simulink model "Sri_Lanka_S_FINAL_set_points"  (R2024a)
settings: Solver=ode15s  StartTime=0.0  StopTime=600  MaxStep=0.01  RelTol=1e-3
StartFcn:
  | Pref_Set_LAK
  | Pref_set_samanala
  | Pref_Set_UTH
  | Pref_Set_RTB
  | Pref_Set_BWT
  | Pref_Set_UKU
  | Pref_Set_SOBA_GT
  | Pref_Set_SOBA_ST
  | Pref_Set_NLX
  | Pref_Set_YUGA
  | Pref_Set_POL
  | Pref_Set_SOBA_GT
  | Pref_Set_CAN
  | Pref_Set_WIM
  | Pref_Set_BRO
  | Pref_Set_UMA
  | Pref_Set_KUK
  | Pref_Set_VIC
  | Pref_Set_KOT
  | Pref_Set_UKT
  | Pref_Set_BAR
  | Pref_set_KEL_UNIT1
  | Pref_set_KEL_UNIT2
  | Pref_set_KEL_UNIT3
  | Pref_Set_OLX_1
  | Pref_Set_OLX_2
  | Pref_Set_UnitA
  | Pref_Set_UnitB
undefined symbols (not defined in the file): BAR_R, BAR_T_ACT, BAR_Unit_S_nom, BRO_R_P, BRO_R_T, BRO_T_G, BRO_T_R, BRO_T_W, BRO_Unit_S_nom, BWT_R_P, BWT_R_T, BWT_T_R, BWT_T_W, BWT_Unit_S_nom, CAN_R_P, CAN_R_T, CAN_T_G, CAN_T_R, CAN_T_W, CAN_Unit_S_nom, D_T, f_base, H_eq, KEL_CC_F_GT, KEL_CC_F_ST, KEL_CC_T_HRSG, KEL_R, KEL_T_CH, KEL_UNIT1_S_nom, KEL_UNIT2_S_nom, KEL_UNIT3_S_nom, KOT_R_P, KOT_R_T, KOT_T_R, KOT_T_W, KOT_Unit_S_nom, KUK_R_P, KUK_R_T, KUK_T_R, KUK_T_W, KUK_Unit_S_nom, LAK_R, LAK_S_nom, LAU_R, LAU_T_FILT, LAU_T_INV, LAU_Unit_S_nom, MAD_R, MAD_T_FILT, MAD_T_INV, MAD_Unit_S_nom, MAN_K_vir, MAN_T_FILT, MAN_T_INV, MAN_Unit_S_nom, NLX_R_P, NLX_R_T, NLX_T_G, NLX_T_R, NLX_T_W ... (+122)
settings Model: Creator=munas  LastModifiedBy=DIMUTHU

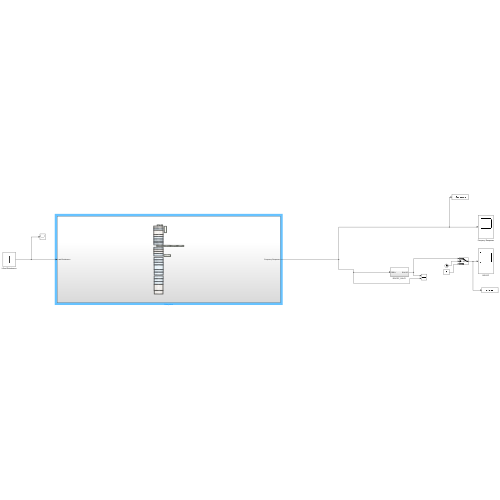
[thumbnail: Simulink's stored preview of the top-level diagram]
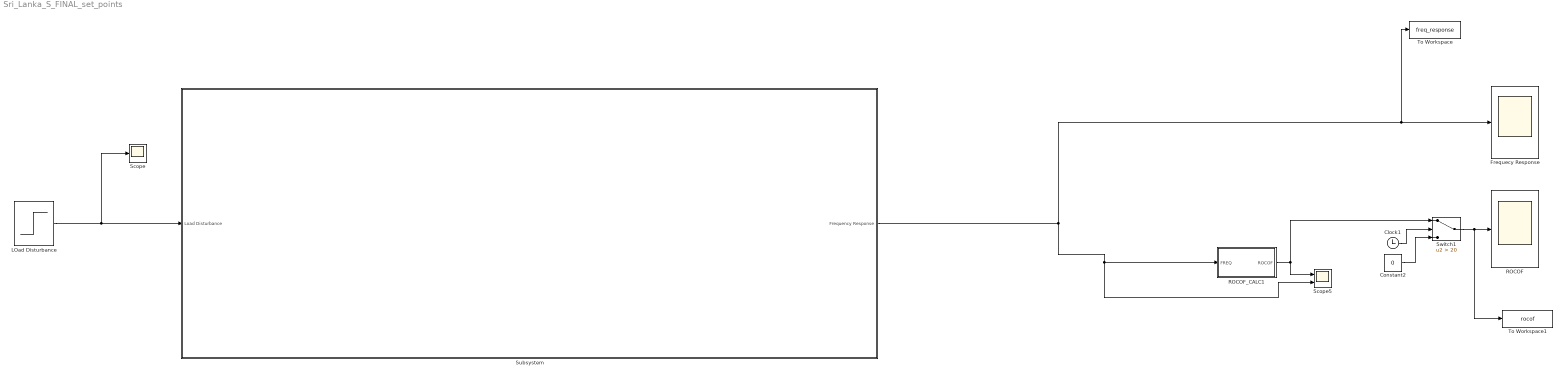
== system Sri_Lanka_S_FINAL_set_points ==
  Clock1 : Clock
  Constant2 : Constant  Value=0
  Frequecy Response : Scope
  LOad Disturbance : Step  Time=t_dist  After=0.05  SampleTime=0
  ROCOF : Scope
  ROCOF_CALC1 : Subsystem
  Scope : Scope
  Scope5 : Scope  NumInputPorts=2
  Subsystem : Subsystem
  Switch1 : Switch  Criteria=u2 > Threshold  Threshold=20  SaturateOnIntegerOverflow=off  InputSameDT=off
  To Workspace : ToWorkspace  VariableName=freq_response  SaveFormat=Timeseries  SampleTime=-1
  To Workspace1 : ToWorkspace  VariableName=rocof  SaveFormat=Timeseries  SampleTime=-1
  wires:
  LOad Disturbance/1 -> Subsystem/1(Load Disturbance), Scope/1
  Subsystem/1(Frequency Response) -> Scope5/2, ROCOF_CALC1/1(FREQ), To Workspace/1, Frequecy Response/1
  Constant2/1 -> Switch1/3
  Switch1/1 -> To Workspace1/1, ROCOF/1
  Clock1/1 -> Switch1/2
  ROCOF_CALC1/1(ROCOF) -> Switch1/1, Scope5/1

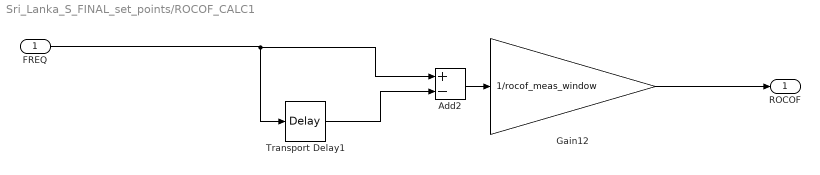
== system Sri_Lanka_S_FINAL_set_points/ROCOF_CALC1 ==
  FREQ : Inport
  Add2 : Sum  Inputs=+-
  Gain12 : Gain  Gain=1/rocof_meas_window
  Transport Delay1 : TransportDelay  DelayTime=rocof_meas_window  InitialOutput=50
  ROCOF : Outport
  wires:
  Transport Delay1/1 -> Add2/2
  Gain12/1 -> ROCOF/1
  Add2/1 -> Gain12/1
  FREQ/1 -> Add2/1, Transport Delay1/1

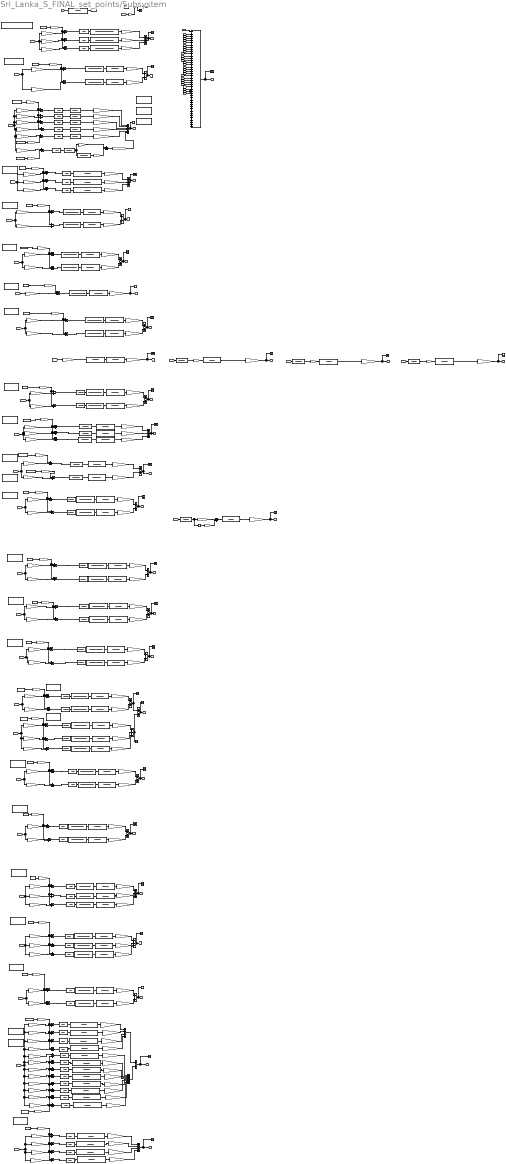
== system Sri_Lanka_S_FINAL_set_points/Subsystem ==
  note: NAYANAJITH
  note: Dinitha
  note: [Steam Turbine Path: 33%]
  note: [Gas Turbine Path: 67%]
  note: SAMANALAWEWA
  note: GRID BLOCK
  note: SUMMING BLOCK
  note: To convert to the frequency
  note: LAKVIJAYA
  note: KELANITISSA
  note: Uthuru Janani plant
  note: RANDENIGALA
  note: RANTAMBE
  note: BOWATENNA
  note: UKUWELA
  note: THAMBAPAVANI WIND FARM: 100 MW
  note: Yugadhanavi GT and ST
  note: New LAXAPANA
  note: Sobadhanavi ST and GT
  note: Polpitiya Plant
  note: Canyon Plant
  note: Wimalasurendra Plant
  note: Kukuleganga Plant
  note: Uma Oya Plant
  note: Old Laxapana Plant
  note: Broadland Plant
  note: Hashan
  note: ANUTHTHARA
  note: Victoria Plant
  note: Upper Kotmale Plant
  note: Kotmale Plant
  note: Colombo Port Barge Plant
  note: Sapugaskanda Plant
  note: Maduru Oya Solar PV subsystem
  note: LAUGFS Hambantota Solar Power Plant
  note: Solar One CeylonSolar Farm
  note: Uppudaluwa Wind Farm
  Load Disturbance : Inport
  " " : TransferFcn  Denominator=[2*H_eq D_T]
  Actuator Delay : TransferFcn  Denominator="[UTH_T_ACT  1]"
  Actuator Delay1 : TransferFcn  Denominator="[UTH_T_ACT  1]"
  Actuator Delay{3..13,15} (12 alike) : TransferFcn  Denominator="[SAP_T_ACT  1]"
  Actuator Delay{14,16..18} (4 alike) : TransferFcn  Denominator="[BAR_T_ACT  1]"
  Actuator Delay2 : TransferFcn  Denominator="[UTH_T_ACT  1]"
  Add{,4,8,13,20..21} (6 alike) : Sum  Inputs=+++
  Add1 : Sum  Inputs=-+++++++++++++++++++++++++++++++++++++++++++
  Add{2,5..7,9..12,14..19,22,25,27..96} (86 alike) : Sum
  Add23 : Sum  Inputs=++++
  Add24 : Sum  Inputs=++++++++
  Add26 : Sum  Inputs=++++
  Add3 : Sum  Inputs=++++++
  Base Scaling Gain : Gain  Gain=SAM_Unit_S_nom / S_base_sys
  Base Scaling Gain GT : Gain  Gain=YUGA_GT_S_nom / S_base_sys
  Base Scaling Gain GT1 : Gain  Gain=YUGA_GT_S_nom / S_base_sys
  Base Scaling Gain GT2 : Gain  Gain=SOBA_GT_S_nom / S_base_sys
  Base Scaling Gain1 : Gain  Gain=SAM_Unit_S_nom / S_base_sys
  Base Scaling Gain10 : Gain  Gain=RTB_Unit_S_nom / S_base_sys
  Base Scaling Gain11 : Gain  Gain=UKU_Unit_S_nom / S_base_sys
  Base Scaling Gain12 : Gain  Gain=BWT_Unit_S_nom / S_base_sys
  Base Scaling Gain13 : Gain  Gain=UKU_Unit_S_nom / S_base_sys
  Base Scaling Gain14 : Gain  Gain=MAN_Unit_S_nom / S_base_sys
  Base Scaling Gain15 : Gain  Gain=SOBA_ST_S_nom/S_base_sys
  Base Scaling Gain16 : Gain  Gain=YUGA_ST_S_nom/S_base_sys
  Base Scaling Gain17 : Gain  Gain=NLX_Unit_S_nom / S_base_sys
  Base Scaling Gain18 : Gain  Gain=NLX_Unit_S_nom / S_base_sys
  Base Scaling Gain19 : Gain  Gain=POL_Unit_S_nom / S_base_sys
  Base Scaling Gain2 : Gain  Gain=RTB_Unit_S_nom / S_base_sys
  Base Scaling Gain20 : Gain  Gain=POL_Unit_S_nom / S_base_sys
  Base Scaling Gain21 : Gain  Gain=WIM_Unit_S_nom / S_base_sys
  Base Scaling Gain22 : Gain  Gain=WIM_Unit_S_nom / S_base_sys
  Base Scaling Gain23 : Gain  Gain=BRO_Unit_S_nom / S_base_sys
  Base Scaling Gain24 : Gain  Gain=BRO_Unit_S_nom / S_base_sys
  Base Scaling Gain25 : Gain  Gain=OLX_Unit_S_nom_1 / S_base_sys
  Base Scaling Gain26 : Gain  Gain=OLX_Unit_S_nom_1 / S_base_sys
  Base Scaling Gain27 : Gain  Gain=OLX_Unit_S_nom_2 / S_base_sys
  Base Scaling Gain28 : Gain  Gain=OLX_Unit_S_nom_2 / S_base_sys
  Base Scaling Gain29 : Gain  Gain=OLX_Unit_S_nom_2 / S_base_sys
  Base Scaling Gain{3..6} (4 alike) : Gain  Gain=KEL_UNIT1_S_nom/ S_base_sys
  Base Scaling Gain30 : Gain  Gain=UMA_Unit_S_nom / S_base_sys
  Base Scaling Gain31 : Gain  Gain=UMA_Unit_S_nom / S_base_sys
  Base Scaling Gain32 : Gain  Gain=KUK_Unit_S_nom / S_base_sys
  Base Scaling Gain33 : Gain  Gain=KUK_Unit_S_nom / S_base_sys
  Base Scaling Gain34 : Gain  Gain=CAN_Unit_S_nom / S_base_sys
  Base Scaling Gain35 : Gain  Gain=CAN_Unit_S_nom / S_base_sys
  Base Scaling Gain36 : Gain  Gain=VIC_Unit_S_nom / S_base_sys
  Base Scaling Gain37 : Gain  Gain=VIC_Unit_S_nom / S_base_sys
  Base Scaling Gain38 : Gain  Gain=VIC_Unit_S_nom / S_base_sys
  Base Scaling Gain39 : Gain  Gain=KOT_Unit_S_nom / S_base_sys
  Base Scaling Gain40 : Gain  Gain=KOT_Unit_S_nom / S_base_sys
  Base Scaling Gain41 : Gain  Gain=UKT_Unit_S_nom / S_base_sys
  Base Scaling Gain42 : Gain  Gain=UKT_Unit_S_nom / S_base_sys
  Base Scaling Gain43 : Gain  Gain=KOT_Unit_S_nom / S_base_sys
  Base Scaling Gain44 : Gain  Gain=MAD_Unit_S_nom / S_base_sys
  Base Scaling Gain45 : Gain  Gain=LAU_Unit_S_nom / S_base_sys
  Base Scaling Gain46 : Gain  Gain=SOC_Unit_S_nom / S_base_sys
  Base Scaling Gain47 : Gain  Gain=UPP_Unit_S_nom / S_base_sys
  Base Scaling Gain7 : Gain  Gain=KEL_UNIT2_S_nom/ S_base_sys
  Base Scaling Gain8 : Gain  Gain=RAN_Unit_S_nom / S_base_sys
  Base Scaling Gain9 : Gain  Gain=RAN_Unit_S_nom / S_base_sys
  Combustr : TransferFcn  Denominator="[KEL_T_CH  1]"
  Constant : Constant  Value=f_base
  Constant1 : Constant  Value=Pref_set_samanala
  Constant10 : Constant  Value=Pref_Set_SOBA_GT
  Constant11 : Constant  Value=Pref_Set_POL
  Constant12 : Constant  Value=Pref_Set_CAN
  Constant13 : Constant  Value=Pref_Set_WIM
  Constant14 : Constant  Value=Pref_Set_BRO
  Constant15 : Constant  Value=Pref_Set_UMA
  Constant16 : Constant  Value=Pref_Set_KUK
  Constant17 : Constant  Value=Pref_Set_VIC
  Constant18 : Constant  Value=Pref_Set_KOT
  Constant19 : Constant  Value=Pref_Set_UKT
  Constant2 : Constant  Value=Pref_Set_LAK
  Constant20 : Constant  Value=Pref_Set_BAR
  Constant21 : Constant  Value=Pref_Set_SOBA_ST
  Constant22 : Constant  Value=Pref_set_KEL_UNIT1
  Constant23 : Constant  Value=Pref_set_KEL_UNIT2
  Constant24 : Constant  Value=Pref_set_KEL_UNIT3
  Constant25 : Constant  Value=Pref_Set_OLX_1
  Constant26 : Constant  Value=Pref_Set_OLX_2
  Constant27 : Constant  Value=Pref_Set_UnitA
  Constant28 : Constant  Value=Pref_Set_UnitB
  Constant3 : Constant  Value=Pref_Set_UTH
  Constant4 : Constant  Value=Pref_Set_RAN
  Constant5 : Constant  Value=Pref_Set_RTB
  Constant6 : Constant  Value=Pref_Set_BWT
  Constant7 : Constant  Value=Pref_Set_UKU
  Constant8 : Constant  Value=Pref_Set_NLX
  Constant9 : Constant  Value=Pref_Set_YUGA
  Derivative : Derivative
  Gain : Gain  Gain=1 / MAD_R
  Gain1 : Gain  Gain=KEL_CC_F_ST
  Gain{8..35} (28 alike) : Gain  Gain=1e6/S_base_sys
  Gain2 : Gain  Gain=KEL_UNIT3_S_nom/ S_base_sys
  Gain3 : Gain  Gain=f_base
  Gain4 : Gain  Gain=1 / LAU_R
  Gain5 : Gain  Gain=1 / SOC_R
  Gain6 : Gain  Gain=1 / UPP_R_P
  Gain7 : Gain  Gain=UPP_K_vir
  Governer{,1..13} (14 alike) : TransferFcn  Denominator=[T_G 1]
  Governer {1..2,7,9,11,13,15,17..19,30..33,35..46} (26 alike) : TransferFcn  Denominator=[T_G 1]
  Governer {8,10,12,14,16} (5 alike) : TransferFcn  Denominator="[KEL_T_CH  1]"
  Governer 20 : TransferFcn  Denominator=[CAN_T_G 1]
  Governer 21 : TransferFcn  Denominator="[WIM_T_G  1]"
  Governer 22 : TransferFcn  Denominator="[WIM_T_G  1]"
  Governer 23 : TransferFcn  Denominator="[BRO_T_G  1]"
  Governer 24 : TransferFcn  Denominator="[BRO_T_G  1]"
  Governer {25..29} (5 alike) : TransferFcn  Denominator="[OLX_T_G  1]"
  Governer 3 : TransferFcn  Denominator=[POL_T_G 1]
  Governer 34 : TransferFcn  Denominator="[CAN_T_G  1]"
  Governer 4 : TransferFcn  Denominator=[POL_T_G 1]
  Governer 5 : TransferFcn  Denominator=[NLX_T_G 1]
  Governer 6 : TransferFcn  Denominator=[NLX_T_G 1]
  Governer GT : TransferFcn  Denominator=[YUGA_GT_T_G 1]
  Governer GT1 : TransferFcn  Denominator=[YUGA_GT_T_G 1]
  Governer GT2 : TransferFcn  Denominator=[SOBA_GT_T_g 1]
  Governer ST : TransferFcn  Denominator=[YUGA_ST_T_ch 1]
  Governer ST1 : TransferFcn  Denominator=[SOBA_ST_T_ch 1]
  HRSG Delay : TransferFcn  Denominator="[KEL_CC_T_HRSG  1]"
  Inverter Delay : TransferFcn  Denominator="[MAN_T_INV  1]"
  Inverter Delay1 : TransferFcn  Denominator=[MAD_T_INV 1]
  Inverter Delay2 : TransferFcn  Denominator=[LAU_T_INV 1]
  Inverter Delay3 : TransferFcn  Denominator=[SOC_T_INV 1]
  Inverter Delay4 : TransferFcn  Denominator=[UPP_T_INV 1]
  PLL Filter : TransferFcn  Denominator=[LAU_T_FILT 1]
  PLL Filter1 : TransferFcn  Denominator=[SOC_T_FILT 1]
  PURE DROOP : Gain  Gain=-1/LAK_R
  PURE DROOP GT : Gain  Gain=-1/YUGA_GT_R
  PURE DROOP GT1 : Gain  Gain=-1/YUGA_GT_R
  PURE DROOP GT2 : Gain  Gain=-1/SOBA_GT_R
  PURE DROOP ST : Gain  Gain=-1/YUGA_ST_R
  PURE DROOP ST1 : Gain  Gain=-1/SOBA_ST_R
  PURE DROOP1 : Gain  Gain=-1/LAK_R
  PURE DROOP{6..11} (6 alike) : Gain  Gain=-1/KEL_R
  PURE DROOP12 : Gain  Gain=-1/UTH_R
  PURE DROOP13 : Gain  Gain=-1/UTH_R
  PURE DROOP14 : Gain  Gain=-1/UTH_R
  PURE DROOP15 : Gain  Gain=-1/RAN_R_P
  PURE DROOP16 : Gain  Gain=-1/RAN_R_P
  PURE DROOP17 : Gain  Gain=-1/RTB_R_P
  PURE DROOP18 : Gain  Gain=-1/UKU_R_P
  PURE DROOP19 : Gain  Gain=-1/BWT_R_P
  PURE DROOP2 : Gain  Gain=-1/LAK_R
  PURE DROOP20 : Gain  Gain=-1/UKU_R_P
  PURE DROOP21 : Gain  Gain=-1/BWT_R_P
  PURE DROOP22 : Gain  Gain=-1/NLX_R_P
  PURE DROOP23 : Gain  Gain=-1/NLX_R_P
  PURE DROOP24 : Gain  Gain=-1/POL_R_P
  PURE DROOP25 : Gain  Gain=-1/POL_R_P
  PURE DROOP26 : Gain  Gain=-1/CAN_R_P
  PURE DROOP27 : Gain  Gain=-1/WIM_R_P
  PURE DROOP28 : Gain  Gain=-1/WIM_R_P
  PURE DROOP29 : Gain  Gain=-1/BRO_R_P
  PURE DROOP3 : Gain  Gain=-1/SAM_R_P
  PURE DROOP30 : Gain  Gain=-1/BRO_R_P
  PURE DROOP{31..35} (5 alike) : Gain  Gain=-1/OLX_R_P
  PURE DROOP36 : Gain  Gain=-1/UMA_R_P
  PURE DROOP37 : Gain  Gain=-1/UMA_R_P
  PURE DROOP38 : Gain  Gain=-1/KUK_R_P
  PURE DROOP39 : Gain  Gain=-1/KUK_R_P
  PURE DROOP4 : Gain  Gain=-1/SAM_R_P
  PURE DROOP40 : Gain  Gain=-1/CAN_R_P
  PURE DROOP41 : Gain  Gain=-1/VIC_R_P
  PURE DROOP42 : Gain  Gain=-1/VIC_R_P
  PURE DROOP43 : Gain  Gain=-1/VIC_R_P
  PURE DROOP44 : Gain  Gain=-1/KOT_R_P
  PURE DROOP45 : Gain  Gain=-1/KOT_R_P
  PURE DROOP46 : Gain  Gain=-1/UKT_R_P
  PURE DROOP47 : Gain  Gain=-1/UKT_R_P
  PURE DROOP48 : Gain  Gain=-1/KOT_R_P
  PURE DROOP{49..60} (12 alike) : Gain  Gain=-1/SAP_R
  PURE DROOP5 : Gain  Gain=-1/RTB_R_P
  PURE DROOP{61..64} (4 alike) : Gain  Gain=-1/BAR_R
  Scaling : Sum
  Scaling 1 : Gain  Gain=LAK_S_nom / S_base_sys
  Scaling {7..10} (4 alike) : Gain  Gain=SAP_A_Unit_S_nom / S_base_sys
  Scaling {11..18} (8 alike) : Gain  Gain=SAP_B_Unit_S_nom / S_base_sys
  Scaling {19..22} (4 alike) : Gain  Gain=BAR_Unit_S_nom / S_base_sys
  Scaling 2 : Gain  Gain=LAK_S_nom / S_base_sys
  Scaling 3 : Gain  Gain=LAK_S_nom / S_base_sys
  Scaling 4 : Gain  Gain=UTH_Unit_S_nom / S_base_sys
  Scaling 5 : Gain  Gain=UTH_Unit_S_nom / S_base_sys
  Scaling 6 : Gain  Gain=UTH_Unit_S_nom / S_base_sys
  Scope{,1..31} (32 alike) : Scope
  Slider : SliderBlock  ScaleMax=300
  Slider1 : SliderBlock  ScaleMax=60
  Slider10 : SliderBlock  ScaleMax=130
  Slider11 : SliderBlock  ScaleMax=45
  Slider12 : SliderBlock  ScaleMax=30
  Slider13 : SliderBlock  ScaleMax=25
  Slider14 : SliderBlock  ScaleMax=17.5
  Slider15 : SliderBlock  ScaleMax=60
  Slider16 : SliderBlock  ScaleMax=40
  Slider17 : SliderBlock  ScaleMax=70
  Slider18 : SliderBlock  ScaleMax=67
  Slider19 : SliderBlock  ScaleMax=83
  Slider2 : SliderBlock  ScaleMax=8
  Slider20 : SliderBlock  ScaleMax=15
  Slider21 : SliderBlock  ScaleMax=20
  Slider22 : SliderBlock  ScaleMax=115
  Slider23 : SliderBlock  ScaleMax=165
  Slider24 : SliderBlock  ScaleMax=12.5
  Slider25 : SliderBlock  ScaleMax=8.33
  Slider26 : SliderBlock  ScaleMax=20
  Slider27 : SliderBlock  ScaleMax=10
  Slider3 : SliderBlock  ScaleMax=63
  Slider4 : SliderBlock  ScaleMax=26
  Slider5 : SliderBlock  ScaleMax=40
  Slider6 : SliderBlock  ScaleMax=20
  Slider7 : SliderBlock  ScaleMax=50
  Slider8 : SliderBlock
  Slider9 : SliderBlock  ScaleMax=220
  Sum : Sum  Inputs=|++
  Synthetic Inertia : TransferFcn  Numerator="[MAN_K_vir  0]"  Denominator="[MAN_T_FILT  1]"
  Transfer Fcn : TransferFcn  Denominator=[MAD_T_FILT 1]
  Transfer Fcn1 : TransferFcn  Denominator=[UPP_T_FILT 1]
  Transient Droop : TransferFcn  Numerator="[SAM_T_R  1]"  Denominator="[SAM_T_R*(SAM_R_T/SAM_R_P)  1]"
  Transient Droop GT : TransferFcn  Denominator="[YUGA_GT_T_t  1]"
  Transient Droop GT1 : TransferFcn  Denominator="[YUGA_GT_T_t  1]"
  Transient Droop GT2 : TransferFcn  Denominator="[SOBA_GT_T_t  1]"
  Transient Droop ST : TransferFcn  Denominator="[YUGA_ST_T_hrsga  1]"
  Transient Droop ST1 : TransferFcn  Denominator="[SOBA_ST_T_hrsga  1]"
  Transient Droop1 : TransferFcn  Numerator="[SAM_T_R  1]"  Denominator="[SAM_T_R*(SAM_R_T/SAM_R_P)  1]"
  Transient Droop10 : TransferFcn  Numerator="[NLX_T_R  1]"  Denominator="[NLX_T_R*(NLX_R_T/NLX_R_P)  1]"
  Transient Droop11 : TransferFcn  Numerator=[POL_T_R 1]  Denominator="[POL_T_R*(POL_R_T/POL_R_P)  1]"
  Transient Droop12 : TransferFcn  Numerator="[POL_T_R  1]"  Denominator="[POL_T_R*(POL_R_T/POL_R_P)  1]"
  Transient Droop13 : TransferFcn  Numerator=[BRO_T_R 1]  Denominator="[BRO_T_R*(BRO_R_T/BRO_R_P)  1]"
  Transient Droop14 : TransferFcn  Numerator=[BRO_T_R 1]  Denominator="[BRO_T_R*(BRO_R_T/BRO_R_P)  1]"
  Transient Droop{15..19} (5 alike) : TransferFcn  Numerator=[OLX_T_R 1]  Denominator="[OLX_T_R*(OLX_R_T/OLX_R_P)  1]"
  Transient Droop2 : TransferFcn  Numerator="[RAN_T_R  1]"  Denominator="[(RAN_R_T / RAN_R_P) * RAN_T_R   1]"
  Transient Droop20 : TransferFcn  Numerator="[UMA_T_R  1]"  Denominator="[UMA_T_R*(UMA_R_T/UMA_R_P)  1]"
  Transient Droop21 : TransferFcn  Numerator="[UMA_T_R  1]"  Denominator="[UMA_T_R*(UMA_R_T/UMA_R_P)  1]"
  Transient Droop22 : TransferFcn  Numerator="[KUK_T_R  1]"  Denominator="[KUK_T_R*(KUK_R_T/KUK_R_P)  1]"
  Transient Droop23 : TransferFcn  Numerator="[KUK_T_R  1]"  Denominator="[KUK_T_R*(KUK_R_T/KUK_R_P)  1]"
  Transient Droop24 : TransferFcn  Numerator=[CAN_T_R 1]  Denominator="[CAN_T_R*(CAN_R_T/CAN_R_P)  1]"
  Transient Droop25 : TransferFcn  Numerator=[CAN_T_R 1]  Denominator="[CAN_T_R*(CAN_R_T/CAN_R_P)  1]"
  Transient Droop26 : TransferFcn  Numerator=[WIM_T_R 1]  Denominator="[WIM_T_R*(WIM_R_T/WIM_R_P)  1]"
  Transient Droop27 : TransferFcn  Numerator=[WIM_T_R 1]  Denominator="[WIM_T_R*(WIM_R_T/WIM_R_P)  1]"
  Transient Droop28 : TransferFcn  Numerator="[VIC_T_R  1]"  Denominator="[VIC_T_R*(VIC_R_T/VIC_R_P)  1]"
  Transient Droop29 : TransferFcn  Numerator="[VIC_T_R  1]"  Denominator="[VIC_T_R*(VIC_R_T/VIC_R_P)  1]"
  Transient Droop3 : TransferFcn  Numerator="[RAN_T_R  1]"  Denominator="[(RAN_R_T / RAN_R_P) * RAN_T_R   1]"
  Transient Droop30 : TransferFcn  Numerator="[VIC_T_R  1]"  Denominator="[VIC_T_R*(VIC_R_T/VIC_R_P)  1]"
  Transient Droop31 : TransferFcn  Numerator="[KOT_T_R  1]"  Denominator="[KOT_T_R*(KOT_R_T/KOT_R_P)  1]"
  Transient Droop32 : TransferFcn  Numerator="[KOT_T_R  1]"  Denominator="[KOT_T_R*(KOT_R_T/KOT_R_P)  1]"
  Transient Droop33 : TransferFcn  Numerator="[UKT_T_R  1]"  Denominator="[UKT_T_R*(UKT_R_T/UKT_R_P)  1]"
  Transient Droop34 : TransferFcn  Numerator="[UKT_T_R  1]"  Denominator="[UKT_T_R*(UKT_R_T/UKT_R_P)  1]"
  Transient Droop35 : TransferFcn  Numerator="[KOT_T_R  1]"  Denominator="[KOT_T_R*(KOT_R_T/KOT_R_P)  1]"
  Transient Droop4 : TransferFcn  Numerator="[RTB_T_R  1]"  Denominator="[(RTB_R_T / RTB_R_P) * RTB_T_R   1]"
  Transient Droop5 : TransferFcn  Numerator="[RTB_T_R  1]"  Denominator="[(RTB_R_T / RTB_R_P) * RTB_T_R   1]"
  Transient Droop6 : TransferFcn  Numerator="[BWT_T_R  1]"  Denominator="[(BWT_R_T / BWT_R_P) * BWT_T_R   1]"
  Transient Droop7 : TransferFcn  Numerator="[UKU_T_R  1]"  Denominator="[(UKU_R_T / UKU_R_P) * UKU_T_R   1]"
  Transient Droop8 : TransferFcn  Numerator="[UKU_T_R  1]"  Denominator="[(UKU_R_T / UKU_R_P) * UKU_T_R   1]"
  Transient Droop9 : TransferFcn  Numerator=[NLX_T_R 1]  Denominator="[NLX_T_R*(NLX_R_T/NLX_R_P)  1]"
  Turbine Dynamics (Reheat) : TransferFcn  Numerator="[RHT_F_HP*RHT_T_RH  1]"  Denominator="[RHT_T_CH*RHT_T_RH  (RHT_T_CH+RHT_T_RH)  1]"
  Turbine Dynamics (Reheat)1 : TransferFcn  Numerator="[RHT_F_HP*RHT_T_RH  1]"  Denominator="[RHT_T_CH*RHT_T_RH  (RHT_T_CH+RHT_T_RH)  1]"
  Turbine Dynamics (Reheat)2 : TransferFcn  Numerator="[RHT_F_HP*RHT_T_RH  1]"  Denominator="[RHT_T_CH*RHT_T_RH  (RHT_T_CH+RHT_T_RH)  1]"
  Water Column : TransferFcn  Numerator="[-SAM_T_W  1]"  Denominator="[0.5*SAM_T_W  1]"
  Water Column1 : TransferFcn  Numerator="[-SAM_T_W  1]"  Denominator="[0.5*SAM_T_W  1]"
  Water Column10 : TransferFcn  Numerator="[-NLX_T_W  1]"  Denominator="[0.5*NLX_T_W  1]"
  Water Column11 : TransferFcn  Numerator="[-POL_T_W  1]"  Denominator="[0.5*POL_T_W  1]"
  Water Column12 : TransferFcn  Numerator="[-POL_T_W  1]"  Denominator="[0.5*POL_T_W  1]"
  Water Column13 : TransferFcn  Numerator="[-BRO_T_W  1]"  Denominator="[0.5*BRO_T_W  1]"
  Water Column14 : TransferFcn  Numerator="[-BRO_T_W  1]"  Denominator="[0.5*BRO_T_W  1]"
  Water Column{15..19} (5 alike) : TransferFcn  Numerator="[-OLX_T_W  1]"  Denominator="[0.5*OLX_T_W  1]"
  Water Column2 : TransferFcn  Numerator="[-RAN_T_W  1]"  Denominator="[0.5 * RAN_T_W   1]"
  Water Column20 : TransferFcn  Numerator="[-UMA_T_W  1]"  Denominator="[0.5*UMA_T_W  1]"
  Water Column21 : TransferFcn  Numerator="[-UMA_T_W  1]"  Denominator="[0.5*UMA_T_W  1]"
  Water Column22 : TransferFcn  Numerator="[-KUK_T_W  1]"  Denominator="[0.5*KUK_T_W  1]"
  Water Column23 : TransferFcn  Numerator="[-KUK_T_W  1]"  Denominator="[0.5*KUK_T_W  1]"
  Water Column24 : TransferFcn  Numerator="[-CAN_T_W  1]"  Denominator="[0.5*CAN_T_W  1]"
  Water Column25 : TransferFcn  Numerator="[-CAN_T_W  1]"  Denominator="[0.5*CAN_T_W  1]"
  Water Column26 : TransferFcn  Numerator="[-WIM_T_W  1]"  Denominator="[0.5*WIM_T_W  1]"
  Water Column27 : TransferFcn  Numerator="[-WIM_T_W  1]"  Denominator="[0.5*WIM_T_W  1]"
  Water Column28 : TransferFcn  Numerator="[-VIC_T_W  1]"  Denominator="[0.5*VIC_T_W  1]"
  Water Column29 : TransferFcn  Numerator="[-VIC_T_W  1]"  Denominator="[0.5*VIC_T_W  1]"
  Water Column3 : TransferFcn  Numerator="[-RAN_T_W  1]"  Denominator="[0.5 * RAN_T_W   1]"
  Water Column30 : TransferFcn  Numerator="[-VIC_T_W  1]"  Denominator="[0.5*VIC_T_W  1]"
  Water Column31 : TransferFcn  Numerator="[-KOT_T_W  1]"  Denominator="[0.5*KOT_T_W  1]"
  Water Column32 : TransferFcn  Numerator="[-KOT_T_W  1]"  Denominator="[0.5*KOT_T_W  1]"
  Water Column33 : TransferFcn  Numerator="[-UKT_T_W  1]"  Denominator="[0.5*UKT_T_W  1]"
  Water Column34 : TransferFcn  Numerator="[-UKT_T_W  1]"  Denominator="[0.5*UKT_T_W  1]"
  Water Column35 : TransferFcn  Numerator="[-KOT_T_W  1]"  Denominator="[0.5*KOT_T_W  1]"
  Water Column4 : TransferFcn  Numerator="[-RTB_T_W  1]"  Denominator="[0.5 * RTB_T_W   1]"
  Water Column5 : TransferFcn  Numerator="[-RTB_T_W  1]"  Denominator="[0.5 * RTB_T_W   1]"
  Water Column6 : TransferFcn  Numerator="[-BWT_T_W  1]"  Denominator="[0.5 * BWT_T_W   1]"
  Water Column7 : TransferFcn  Numerator="[-UKU_T_W  1]"  Denominator="[0.5 * UKU_T_W   1]"
  Water Column8 : TransferFcn  Numerator="[-UKU_T_W  1]"  Denominator="[0.5 * UKU_T_W   1]"
  Water Column9 : TransferFcn  Numerator="[-NLX_T_W  1]"  Denominator="[0.5*NLX_T_W  1]"
  | Gain: F_GT : Gain  Gain=KEL_CC_F_GT
  Frequency Response : Outport
  wires:
  Governer 1/1 -> Turbine Dynamics (Reheat)/1
  Turbine Dynamics (Reheat)/1 -> Scaling 1/1
  Sum/1 -> Scope2/1, Frequency Response/1
  Constant/1 -> Sum/1
  Scaling 1/1 -> Add/1
  Governer 2/1 -> Turbine Dynamics (Reheat)1/1
  Turbine Dynamics (Reheat)1/1 -> Scaling 2/1
  Scaling 2/1 -> Add/2
  Governer/1 -> Turbine Dynamics (Reheat)2/1
  Turbine Dynamics (Reheat)2/1 -> Scaling 3/1
  Scaling 3/1 -> Add/3
  Add/1 -> Scope3/1, [LAK]
  [P_acc] -> " "/1
  " "/1 -> [Rotor_Dev]
  [Rotor_Dev] -> PURE DROOP2/1, PURE DROOP/1, PURE DROOP1/1
  [Rotor_Dev] -> Gain3/1
  [LAK] -> Add1/2
  Add1/1 -> Scope/1, [P_acc]
  Load Disturbance/1 -> Add1/1
  [Rotor_Dev] -> PURE DROOP3/1, PURE DROOP4/1
  Base Scaling Gain/1 -> Add2/1
  Add2/1 -> Scope1/1, [SAM]
  Transient Droop/1 -> Water Column/1
  Water Column/1 -> Base Scaling Gain/1
  Water Column1/1 -> Base Scaling Gain1/1
  Transient Droop1/1 -> Water Column1/1
  Base Scaling Gain1/1 -> Add2/2
  [SAM] -> Add1/3
  Gain3/1 -> Sum/2
  [Rotor_Dev] -> PURE DROOP8/1, PURE DROOP7/1, PURE DROOP6/1, PURE DROOP11/1, PURE DROOP10/1, PURE DROOP9/1
  Governer 7/1 -> Governer 8/1
  Governer 8/1 -> Base Scaling Gain3/1
  Governer 9/1 -> Governer 10/1
  Governer 10/1 -> Base Scaling Gain4/1
  Governer 11/1 -> Governer 12/1
  Governer 12/1 -> Base Scaling Gain5/1
  Governer 13/1 -> Governer 14/1
  Governer 14/1 -> Base Scaling Gain6/1
  Governer 15/1 -> Governer 16/1
  Governer 16/1 -> Base Scaling Gain7/1
  Governer 17/1 -> Combustr/1
  HRSG Delay/1 -> Gain1/1
  Combustr/1 -> HRSG Delay/1, | Gain: F_GT/1
  | Gain: F_GT/1 -> Scaling/1
  Gain1/1 -> Scaling/2
  Scaling/1 -> Gain2/1
  Base Scaling Gain3/1 -> Add3/1
  Base Scaling Gain4/1 -> Add3/2
  Base Scaling Gain5/1 -> Add3/3
  Base Scaling Gain6/1 -> Add3/4
  Base Scaling Gain7/1 -> Add3/5
  Gain2/1 -> Add3/6
  Add3/1 -> Scope9/1, [KEL]
  [KEL] -> Add1/4
  Actuator Delay2/1 -> Scaling 6/1
  Add4/1 -> Scope4/1, [UTH]
  Scaling 6/1 -> Add4/3
  Governer 19/1 -> Actuator Delay1/1
  Governer1/1 -> Actuator Delay2/1
  Scaling 4/1 -> Add4/1
  [Rotor_Dev] -> PURE DROOP14/1, PURE DROOP13/1, PURE DROOP12/1
  Actuator Delay1/1 -> Scaling 5/1
  Governer 18/1 -> Actuator Delay/1
  Scaling 5/1 -> Add4/2
  Actuator Delay/1 -> Scaling 4/1
  [UTH] -> Add1/5
  [Rotor_Dev] -> PURE DROOP16/1, PURE DROOP15/1
  Transient Droop2/1 -> Water Column2/1
  Base Scaling Gain8/1 -> Add5/1
  Water Column2/1 -> Base Scaling Gain8/1
  Add5/1 -> Scope5/1, [RAN]
  Transient Droop3/1 -> Water Column3/1
  Water Column3/1 -> Base Scaling Gain9/1
  Base Scaling Gain9/1 -> Add5/2
  [RAN] -> Add1/6
  Add6/1 -> Scope6/1, [RTB]
  [Rotor_Dev] -> PURE DROOP17/1, PURE DROOP5/1
  Water Column4/1 -> Base Scaling Gain2/1
  Base Scaling Gain2/1 -> Add6/1
  Base Scaling Gain10/1 -> Add6/2
  Transient Droop4/1 -> Water Column4/1
  [RTB] -> Add1/7
  Transient Droop5/1 -> Water Column5/1
  Water Column5/1 -> Base Scaling Gain10/1
  Transient Droop6/1 -> Water Column6/1
  [Rotor_Dev] -> PURE DROOP19/1
  Water Column6/1 -> Base Scaling Gain12/1
  Base Scaling Gain12/1 -> Scope7/1, [BWT]
  [BWT] -> Add1/8
  Transient Droop7/1 -> Water Column7/1
  Base Scaling Gain13/1 -> Add7/1
  [Rotor_Dev] -> PURE DROOP18/1, PURE DROOP20/1
  Water Column7/1 -> Base Scaling Gain13/1
  Add7/1 -> Scope8/1, [UKU]
  Base Scaling Gain11/1 -> Add7/2
  Water Column8/1 -> Base Scaling Gain11/1
  Transient Droop8/1 -> Water Column8/1
  [UKU] -> Add1/9
  Base Scaling Gain14/1 -> Scope10/1, [MAN]
  Inverter Delay/1 -> Base Scaling Gain14/1
  [Rotor_Dev] -> PURE DROOP21/1
  PURE DROOP21/1 -> Synthetic Inertia/1
  Synthetic Inertia/1 -> Inverter Delay/1
  [MAN] -> Add1/10
  Water Column10/1 -> Base Scaling Gain18/1
  Water Column11/1 -> Base Scaling Gain19/1
  Governer 6/1 -> Transient Droop10/1
  Base Scaling Gain GT2/1 -> Add9/1
  Base Scaling Gain17/1 -> Add10/1
  Transient Droop10/1 -> Water Column10/1
  Governer GT2/1 -> Transient Droop GT2/1
  Add9/1 -> Scope12/1, [SOBA]
  Transient Droop9/1 -> Water Column9/1
  Base Scaling Gain GT/1 -> Add8/1
  Base Scaling Gain15/1 -> Add9/2
  Governer ST/1 -> Transient Droop ST/1
  Transient Droop GT/1 -> Base Scaling Gain GT/1
  [Rotor_Dev] -> PURE DROOP ST/1, PURE DROOP GT1/1, PURE DROOP GT/1
  Base Scaling Gain GT1/1 -> Add8/2
  Transient Droop GT1/1 -> Base Scaling Gain GT1/1
  Governer 3/1 -> Transient Droop11/1
  [Rotor_Dev] -> PURE DROOP25/1, PURE DROOP24/1
  Governer 5/1 -> Transient Droop9/1
  Base Scaling Gain19/1 -> Add11/1
  Base Scaling Gain18/1 -> Add10/2
  Transient Droop GT2/1 -> Base Scaling Gain GT2/1
  Governer GT/1 -> Transient Droop GT/1
  Add8/1 -> Scope11/1, [YUGA]
  Transient Droop ST/1 -> Base Scaling Gain16/1
  Governer 4/1 -> Transient Droop12/1
  [Rotor_Dev] -> PURE DROOP23/1, PURE DROOP22/1
  [Rotor_Dev] -> PURE DROOP ST1/1, PURE DROOP GT2/1
  Add11/1 -> Scope14/1, [POL]
  Base Scaling Gain20/1 -> Add11/2
  Transient Droop ST1/1 -> Base Scaling Gain15/1
  Transient Droop11/1 -> Water Column11/1
  Governer GT1/1 -> Transient Droop GT1/1
  Base Scaling Gain16/1 -> Add8/3
  Add10/1 -> Scope13/1, [NLX]
  Water Column9/1 -> Base Scaling Gain17/1
  Water Column12/1 -> Base Scaling Gain20/1
  Governer ST1/1 -> Transient Droop ST1/1
  Transient Droop12/1 -> Water Column12/1
  [NLX] -> Add1/13
  [YUGA] -> Add1/12
  [SOBA] -> Add1/11
  [POL] -> Add1/14
  Base Scaling Gain33/1 -> Add16/2
  Transient Droop21/1 -> Water Column21/1
  Add14/1 -> Scope18/1, [OLX]
  Governer 29/1 -> Transient Droop19/1
  [Rotor_Dev] -> PURE DROOP39/1, PURE DROOP38/1
  Base Scaling Gain21/1 -> Add18/1
  Governer 27/1 -> Transient Droop18/1
  Base Scaling Gain24/1 -> Add19/2
  Governer 33/1 -> Transient Droop23/1
  Base Scaling Gain32/1 -> Add16/1
  Transient Droop20/1 -> Water Column20/1
  Water Column15/1 -> Base Scaling Gain25/1
  Water Column23/1 -> Base Scaling Gain33/1
  Base Scaling Gain31/1 -> Add15/2
  Governer 26/1 -> Transient Droop15/1
  Base Scaling Gain30/1 -> Add15/1
  Water Column21/1 -> Base Scaling Gain31/1
  Base Scaling Gain28/1 -> Add13/2
  Add15/1 -> Scope19/1, [UMA]
  Governer 30/1 -> Transient Droop20/1
  [Rotor_Dev] -> PURE DROOP31/1, PURE DROOP32/1
  Water Column13/1 -> Base Scaling Gain23/1
  Governer 28/1 -> Transient Droop17/1
  [Rotor_Dev] -> PURE DROOP26/1, PURE DROOP40/1
  [Rotor_Dev] -> PURE DROOP29/1, PURE DROOP30/1
  Transient Droop19/1 -> Water Column19/1
  Add18/1 -> Scope22/1, [WIM]
  Water Column18/1 -> Base Scaling Gain28/1
  Add13/1 -> Add14/2, Scope17/1
  Water Column22/1 -> Base Scaling Gain32/1
  Transient Droop14/1 -> Water Column14/1
  Governer 24/1 -> Transient Droop13/1
  Transient Droop15/1 -> Water Column15/1
  Base Scaling Gain27/1 -> Add13/1
  [Rotor_Dev] -> PURE DROOP35/1, PURE DROOP33/1, PURE DROOP34/1
  Water Column24/1 -> Base Scaling Gain34/1
  Transient Droop22/1 -> Water Column22/1
  Water Column16/1 -> Base Scaling Gain26/1
  Transient Droop18/1 -> Water Column18/1
  Governer 25/1 -> Transient Droop16/1
  Transient Droop17/1 -> Water Column17/1
  Water Column14/1 -> Base Scaling Gain24/1
  Base Scaling Gain22/1 -> Add18/2
  [Rotor_Dev] -> PURE DROOP27/1, PURE DROOP28/1
  Governer 21/1 -> Transient Droop27/1
  Transient Droop16/1 -> Water Column16/1
  Base Scaling Gain29/1 -> Add13/3
  Transient Droop26/1 -> Water Column26/1
  Governer 23/1 -> Transient Droop14/1
  Transient Droop27/1 -> Water Column27/1
  [Rotor_Dev] -> PURE DROOP37/1, PURE DROOP36/1
  Base Scaling Gain23/1 -> Add19/1
  Transient Droop13/1 -> Water Column13/1
  Water Column25/1 -> Base Scaling Gain35/1
  Governer 20/1 -> Transient Droop25/1
  Add19/1 -> Scope15/1, [BRO]
  Transient Droop25/1 -> Water Column25/1
  Water Column17/1 -> Base Scaling Gain27/1
  Base Scaling Gain34/1 -> Add17/1
  Governer 34/1 -> Transient Droop24/1
  Transient Droop24/1 -> Water Column24/1
  Governer 22/1 -> Transient Droop26/1
  Base Scaling Gain26/1 -> Add12/2
  Add16/1 -> Scope20/1, [KUK]
  Base Scaling Gain35/1 -> Add17/2
  Water Column26/1 -> Base Scaling Gain21/1
  Add17/1 -> Scope21/1, [CAN]
  Add12/1 -> Add14/1, Scope16/1
  Governer 32/1 -> Transient Droop22/1
  Governer 31/1 -> Transient Droop21/1
  Water Column27/1 -> Base Scaling Gain22/1
  Water Column20/1 -> Base Scaling Gain30/1
  Transient Droop23/1 -> Water Column23/1
  Water Column19/1 -> Base Scaling Gain29/1
  Base Scaling Gain25/1 -> Add12/1
  [BRO] -> Add1/17
  [WIM] -> Add1/16
  [UMA] -> Add1/19
  [CAN] -> Add1/15
  [KUK] -> Add1/20
  [OLX] -> Add1/18
  Scaling 22/1 -> Add26/4
  Governer13/1 -> Actuator Delay17/1
  Base Scaling Gain37/1 -> Add20/2
  Actuator Delay5/1 -> Scaling 15/1
  Actuator Delay15/1 -> Scaling 16/1
  Actuator Delay14/1 -> Scaling 19/1
  [Rotor_Dev] -> PURE DROOP43/1, PURE DROOP41/1, PURE DROOP42/1
  Governer 35/1 -> Transient Droop28/1
  Scaling 20/1 -> Add26/1
  Scaling 14/1 -> Add24/3
  Water Column33/1 -> Base Scaling Gain41/1
  Water Column32/1 -> Base Scaling Gain40/1
  Scaling 18/1 -> Add24/6
  Scaling 11/1 -> Add24/1
  Water Column30/1 -> Base Scaling Gain38/1
  Actuator Delay10/1 -> Scaling 17/1
  Actuator Delay7/1 -> Scaling 12/1
  Actuator Delay8/1 -> Scaling 13/1
  Scaling 7/1 -> Add23/1
  Scaling 19/1 -> Add26/2
  Actuator Delay4/1 -> Scaling 11/1
  Add22/1 -> Scope25/1, [UKT]
  Scaling 9/1 -> Add23/3
  [Rotor_Dev] -> PURE DROOP48/1, PURE DROOP45/1, PURE DROOP44/1
  Actuator Delay11/1 -> Scaling 9/1
  Actuator Delay12/1 -> Scaling 8/1
  Actuator Delay13/1 -> Scaling 10/1
  Governer5/1 -> Actuator Delay5/1
  Base Scaling Gain40/1 -> Add21/2
  Governer3/1 -> Actuator Delay4/1
  Governer4/1 -> Actuator Delay13/1
  Governer10/1 -> Actuator Delay10/1
  Governer9/1 -> Actuator Delay9/1
  Governer6/1 -> Actuator Delay6/1
  Governer 43/1 -> Actuator Delay3/1
  [Rotor_Dev] -> PURE DROOP53/1, PURE DROOP52/1, PURE DROOP49/1, PURE DROOP50/1, PURE DROOP51/1, PURE DROOP55/1, PURE DROOP60/1, PURE DROOP59/1, PURE DROOP58/1, PURE DROOP57/1, PURE DROOP56/1, PURE DROOP54/1
  Governer2/1 -> Actuator Delay11/1
  Scaling 8/1 -> Add23/2
  Add26/1 -> Scope26/1, [BAR]
  Actuator Delay3/1 -> Scaling 7/1
  Base Scaling Gain41/1 -> Add22/1
  Governer 44/1 -> Actuator Delay12/1
  Base Scaling Gain43/1 -> Add21/3
  Scaling 10/1 -> Add23/4
  Base Scaling Gain39/1 -> Add21/1
  Transient Droop32/1 -> Water Column32/1
  Water Column35/1 -> Base Scaling Gain43/1
  Governer 42/1 -> Transient Droop35/1
  Water Column31/1 -> Base Scaling Gain39/1
  Transient Droop35/1 -> Water Column35/1
  Transient Droop34/1 -> Water Column34/1
  Governer 39/1 -> Transient Droop32/1
  Governer 40/1 -> Transient Droop33/1
  Transient Droop31/1 -> Water Column31/1
  Water Column29/1 -> Base Scaling Gain37/1
  Governer 38/1 -> Transient Droop31/1
  Base Scaling Gain42/1 -> Add22/2
  Transient Droop29/1 -> Water Column29/1
  Governer7/1 -> Actuator Delay7/1
  Base Scaling Gain38/1 -> Add20/3
  Add20/1 -> Scope23/1, [VIC]
  Water Column28/1 -> Base Scaling Gain36/1
  [Rotor_Dev] -> PURE DROOP47/1, PURE DROOP46/1
  Actuator Delay16/1 -> Scaling 21/1
  Actuator Delay17/1 -> Scaling 22/1
  Governer 46/1 -> Actuator Delay14/1
  Base Scaling Gain36/1 -> Add20/1
  Add21/1 -> Scope24/1, [KOT]
  Governer8/1 -> Actuator Delay8/1
  Scaling 13/1 -> Add24/5
  [Rotor_Dev] -> PURE DROOP62/1, PURE DROOP61/1, PURE DROOP63/1, PURE DROOP64/1
  Add25/1 -> Scope27/1, [SAP]
  Governer11/1 -> Actuator Delay15/1
  Governer 45/1 -> Actuator Delay18/1
  Transient Droop30/1 -> Water Column30/1
  Scaling 17/1 -> Add24/7
  Actuator Delay18/1 -> Scaling 20/1
  Governer12/1 -> Actuator Delay16/1
  Transient Droop33/1 -> Water Column33/1
  Governer 36/1 -> Transient Droop29/1
  Scaling 12/1 -> Add24/4
  Add23/1 -> Add25/1
  Governer 41/1 -> Transient Droop34/1
  Scaling 16/1 -> Add24/8
  Scaling 15/1 -> Add24/2
  Actuator Delay9/1 -> Scaling 18/1
  Transient Droop28/1 -> Water Column28/1
  Scaling 21/1 -> Add26/3
  Actuator Delay6/1 -> Scaling 14/1
  Governer 37/1 -> Transient Droop30/1
  Water Column34/1 -> Base Scaling Gain42/1
  Add24/1 -> Add25/2
  [VIC] -> Add1/21
  [UKT] -> Add1/23
  [SAP] -> Add1/24
  [BAR] -> Add1/25
  [KOT] -> Add1/22
  Inverter Delay1/1 -> Base Scaling Gain44/1
  Gain/1 -> Inverter Delay1/1
  Base Scaling Gain44/1 -> Scope28/1, [MAD]
  Transfer Fcn/1 -> Gain/1
  [Rotor_Dev] -> Transfer Fcn/1
  [MAD] -> Add1/26
  [Rotor_Dev] -> PLL Filter/1
  Gain4/1 -> Inverter Delay2/1
  Base Scaling Gain45/1 -> Scope29/1, [LAU]
  PLL Filter/1 -> Gain4/1
  Inverter Delay2/1 -> Base Scaling Gain45/1
  [LAU] -> Add1/27
  PLL Filter1/1 -> Gain5/1
  Base Scaling Gain46/1 -> Scope30/1, [SOC]
  Gain5/1 -> Inverter Delay3/1
  Inverter Delay3/1 -> Base Scaling Gain46/1
  [Rotor_Dev] -> PLL Filter1/1
  [SOC] -> Add1/28
  [Rotor_Dev] -> Transfer Fcn1/1
  Transfer Fcn1/1 -> Derivative/1, Gain6/1
  Inverter Delay4/1 -> Base Scaling Gain47/1
  Base Scaling Gain47/1 -> Scope31/1, [UPP]
  Derivative/1 -> Gain7/1
  Gain7/1 -> Add28/2
  Gain6/1 -> Add28/1
  Add28/1 -> Inverter Delay4/1
  [UPP] -> Add1/29
  Constant2/1 -> Gain8/1
  Add27/1 -> Governer 1/1
  PURE DROOP/1 -> Add27/2
  Add29/1 -> Governer 2/1
  Add30/1 -> Governer/1
  Gain8/1 -> Add27/1, Add29/1, Add30/1
  PURE DROOP1/1 -> Add29/2
  PURE DROOP2/1 -> Add30/2
  Add32/1 -> Transient Droop1/1
  Add31/1 -> Transient Droop/1
  Gain9/1 -> Add31/1, Add32/1
  PURE DROOP3/1 -> Add31/2
  PURE DROOP4/1 -> Add32/2
  Constant1/1 -> Gain9/1
  PURE DROOP14/1 -> Add35/2
  Add35/1 -> Governer1/1
  Add34/1 -> Governer 19/1
  Add33/1 -> Governer 18/1
  Gain10/1 -> Add33/1, Add34/1, Add35/1
  PURE DROOP12/1 -> Add33/2
  PURE DROOP13/1 -> Add34/2
  Constant3/1 -> Gain10/1
  PURE DROOP16/1 -> Add37/2
  Gain11/1 -> Add36/1, Add37/1
  Add37/1 -> Transient Droop3/1
  PURE DROOP15/1 -> Add36/2
  Add36/1 -> Transient Droop2/1
  Constant4/1 -> Gain11/1
  Gain12/1 -> Add38/1, Add39/1
  PURE DROOP5/1 -> Add38/2
  PURE DROOP17/1 -> Add39/2
  Add38/1 -> Transient Droop4/1
  Add39/1 -> Transient Droop5/1
  Add40/1 -> Transient Droop6/1
  Gain13/1 -> Add40/1
  PURE DROOP19/1 -> Add40/2
  Add41/1 -> Transient Droop7/1
  Add42/1 -> Transient Droop8/1
  Gain14/1 -> Add41/1, Add42/1
  PURE DROOP18/1 -> Add42/2
  PURE DROOP20/1 -> Add41/2
  Constant5/1 -> Gain12/1
  Constant6/1 -> Gain13/1
  Constant7/1 -> Gain14/1
  Gain15/1 -> Add43/1, Add44/1
  Gain16/1 -> Add48/1, Add47/1, Add46/1
  Gain17/1 -> Add49/1
  Gain18/1 -> Add52/1, Add53/1
  Gain19/1 -> Add55/1, Add56/1
  Gain20/1 -> Add58/1, Add59/1
  Gain21/1 -> Add61/1, Add62/1
  Gain24/1 -> Add70/1, Add71/1
  Gain25/1 -> Add73/1, Add74/1
  Gain26/1 -> Add76/1, Add77/1, Add78/1
  Gain27/1 -> Add81/1, Add80/1, Add79/1
  Gain28/1 -> Add82/1, Add83/1
  Gain29/1 -> Add86/1, Add87/1, Add45/1, Add85/1
  PURE DROOP22/1 -> Add43/2
  Add43/1 -> Governer 5/1
  Add44/1 -> Governer 6/1
  PURE DROOP23/1 -> Add44/2
  PURE DROOP ST/1 -> Add48/2
  PURE DROOP GT1/1 -> Add47/2
  PURE DROOP GT/1 -> Add46/2
  Add46/1 -> Governer GT/1
  Add47/1 -> Governer GT1/1
  Add48/1 -> Governer ST/1
  PURE DROOP GT2/1 -> Add49/2
  Add49/1 -> Governer GT2/1
  PURE DROOP ST1/1 -> Add50/2
  Add50/1 -> Governer ST1/1
  Add53/1 -> Governer 4/1
  Add52/1 -> Governer 3/1
  PURE DROOP24/1 -> Add52/2
  PURE DROOP25/1 -> Add53/2
  Add56/1 -> Governer 20/1
  Add55/1 -> Governer 34/1
  PURE DROOP26/1 -> Add56/2
  PURE DROOP40/1 -> Add55/2
  Add58/1 -> Governer 22/1
  PURE DROOP28/1 -> Add58/2
  PURE DROOP27/1 -> Add59/2
  Add59/1 -> Governer 21/1
  Add62/1 -> Governer 23/1
  PURE DROOP29/1 -> Add62/2
  Add61/1 -> Governer 24/1
  PURE DROOP30/1 -> Add61/2
  Add70/1 -> Governer 30/1
  Add71/1 -> Governer 31/1
  PURE DROOP36/1 -> Add70/2
  PURE DROOP37/1 -> Add71/2
  Add74/1 -> Governer 33/1
  PURE DROOP39/1 -> Add74/2
  PURE DROOP38/1 -> Add73/2
  Add73/1 -> Governer 32/1
  PURE DROOP43/1 -> Add78/2
  Add78/1 -> Governer 37/1
  Add77/1 -> Governer 36/1
  PURE DROOP42/1 -> Add77/2
  Add76/1 -> Governer 35/1
  PURE DROOP41/1 -> Add76/2
  Add81/1 -> Governer 42/1
  Add80/1 -> Governer 39/1
  Add79/1 -> Governer 38/1
  PURE DROOP44/1 -> Add79/2
  PURE DROOP45/1 -> Add80/2
  PURE DROOP48/1 -> Add81/2
  PURE DROOP46/1 -> Add82/2
  Add82/1 -> Governer 40/1
  Add83/1 -> Governer 41/1
  PURE DROOP47/1 -> Add83/2
  PURE DROOP64/1 -> Add45/2
  PURE DROOP63/1 -> Add87/2
  PURE DROOP62/1 -> Add86/2
  PURE DROOP61/1 -> Add85/2
  Add85/1 -> Governer 45/1
  Add86/1 -> Governer 46/1
  Add87/1 -> Governer12/1
  Add45/1 -> Governer13/1
  Constant8/1 -> Gain15/1
  Constant9/1 -> Gain16/1
  Constant10/1 -> Gain17/1
  Constant11/1 -> Gain18/1
  Constant12/1 -> Gain19/1
  Constant13/1 -> Gain20/1
  Constant14/1 -> Gain21/1
  Constant15/1 -> Gain24/1
  Constant16/1 -> Gain25/1
  Constant17/1 -> Gain26/1
  Constant18/1 -> Gain27/1
  Constant19/1 -> Gain28/1
  Constant20/1 -> Gain29/1
  Constant21/1 -> Gain22/1
  Gain22/1 -> Add50/1
  Gain23/1 -> Add51/1, Add54/1, Add60/1, Add57/1
  PURE DROOP6/1 -> Add51/2
  PURE DROOP7/1 -> Add54/2
  PURE DROOP8/1 -> Add57/2
  PURE DROOP9/1 -> Add60/2
  Add51/1 -> Governer 7/1
  Add54/1 -> Governer 9/1
  Add57/1 -> Governer 11/1
  Add60/1 -> Governer 13/1
  PURE DROOP10/1 -> Add63/1
  Gain30/1 -> Add63/2
  Add63/1 -> Governer 15/1
  PURE DROOP11/1 -> Add64/1
  Gain31/1 -> Add64/2
  Add64/1 -> Governer 17/1
  Constant22/1 -> Gain23/1
  Constant23/1 -> Gain30/1
  Constant24/1 -> Gain31/1
  PURE DROOP31/1 -> Add66/2
  Gain32/1 -> Add65/1, Add66/1
  PURE DROOP32/1 -> Add65/2
  Add65/1 -> Governer 26/1
  Add66/1 -> Governer 25/1
  Gain33/1 -> Add67/1, Add68/1, Add69/1
  PURE DROOP33/1 -> Add68/2
  Add68/1 -> Governer 27/1
  Add69/1 -> Governer 29/1
  PURE DROOP35/1 -> Add69/2
  PURE DROOP34/1 -> Add67/2
  Add67/1 -> Governer 28/1
  Constant25/1 -> Gain32/1
  Constant26/1 -> Gain33/1
  Gain34/1 -> Add84/1, Add88/1, Add75/1, Add72/1
  PURE DROOP49/1 -> Add72/2
  PURE DROOP50/1 -> Add75/2
  PURE DROOP51/1 -> Add84/2
  PURE DROOP52/1 -> Add88/2
  Add72/1 -> Governer 43/1
  Add75/1 -> Governer 44/1
  Add84/1 -> Governer2/1
  Add88/1 -> Governer4/1
  PURE DROOP55/1 -> Add89/1
  PURE DROOP53/1 -> Add90/1
  PURE DROOP54/1 -> Add91/1
  PURE DROOP56/1 -> Add92/1
  PURE DROOP57/1 -> Add93/1
  PURE DROOP58/1 -> Add94/1
  PURE DROOP59/1 -> Add95/1
  PURE DROOP60/1 -> Add96/1
  Gain35/1 -> Add96/2, Add95/2, Add93/2, Add92/2, Add91/2, Add89/2, Add90/2, Add94/2
  Add89/1 -> Governer3/1
  Add90/1 -> Governer5/1
  Add91/1 -> Governer6/1
  Add92/1 -> Governer7/1
  Add93/1 -> Governer8/1
  Add94/1 -> Governer9/1
  Add95/1 -> Governer10/1
  Add96/1 -> Governer11/1
  Constant27/1 -> Gain34/1
  Constant28/1 -> Gain35/1
